simulink model "linearacc"  (R2020a)
settings: Solver=VariableStepAuto  StartTime=0.0  StopTime=10.0  RelTol=1e-3
undefined symbols (not defined in the file): Ax, Ay, Az, g, m
settings Model: Creator=Muni Kumar  LastModifiedBy=Muni Kumar

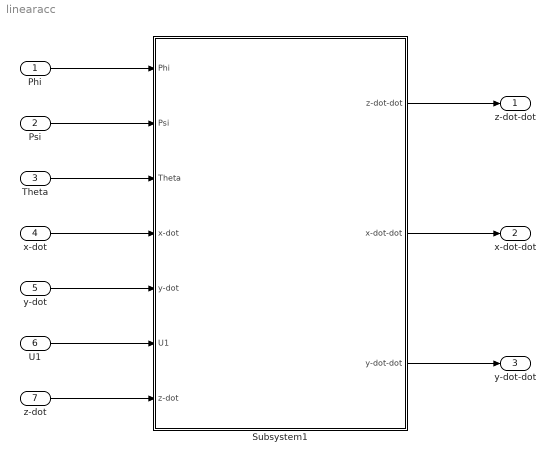
== system linearacc ==
  Phi : Inport
  Psi : Inport  Port=2
  Theta : Inport  Port=3
  x-dot : Inport  Port=4
  y-dot : Inport  Port=5
  U1 : Inport  Port=6
  z-dot : Inport  Port=7
  Subsystem1 : Subsystem
  z-dot-dot : Outport
  x-dot-dot : Outport  Port=2
  y-dot-dot : Outport  Port=3
  wires:
  Phi/1 -> Subsystem1/1(Phi)
  Psi/1 -> Subsystem1/2(Psi)
  Theta/1 -> Subsystem1/3(Theta)
  x-dot/1 -> Subsystem1/4(x-dot)
  U1/1 -> Subsystem1/6(U1)
  z-dot/1 -> Subsystem1/7(z-dot)
  Subsystem1/1(z-dot-dot) -> z-dot-dot/1
  Subsystem1/2(x-dot-dot) -> x-dot-dot/1
  Subsystem1/3(y-dot-dot) -> y-dot-dot/1
  y-dot/1 -> Subsystem1/5(y-dot)

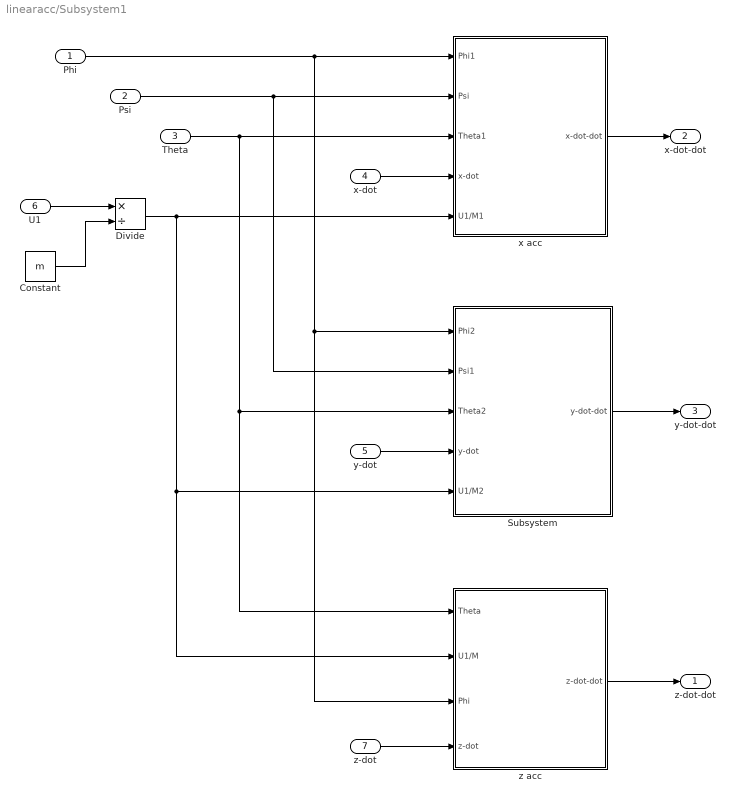
== system linearacc/Subsystem1 ==
  Phi : Inport
  Psi : Inport  Port=2
  Theta : Inport  Port=3
  x-dot : Inport  Port=4
  y-dot : Inport  Port=5
  U1 : Inport  Port=6
  z-dot : Inport  Port=7
  Constant : Constant  Value=m
  Divide : Product  Inputs=*/
  Subsystem : Subsystem
  x acc : Subsystem
  z acc : Subsystem
  z-dot-dot : Outport
  x-dot-dot : Outport  Port=2
  y-dot-dot : Outport  Port=3
  wires:
  Theta/1 -> x acc/3(Theta1), Subsystem/3(Theta2), z acc/1(Theta)
  Phi/1 -> Subsystem/1(Phi2), z acc/3(Phi), x acc/1(Phi1)
  Divide/1 -> Subsystem/5(U1/M2), z acc/2(U1/M), x acc/5(U1/M1)
  y-dot/1 -> Subsystem/4(y-dot)
  Constant/1 -> Divide/2
  Psi/1 -> Subsystem/2(Psi1), x acc/2(Psi)
  z-dot/1 -> z acc/4(z-dot)
  U1/1 -> Divide/1
  x-dot/1 -> x acc/4(x-dot)
  x acc/1(x-dot-dot) -> x-dot-dot/1
  z acc/1(z-dot-dot) -> z-dot-dot/1
  Subsystem/1(y-dot-dot) -> y-dot-dot/1

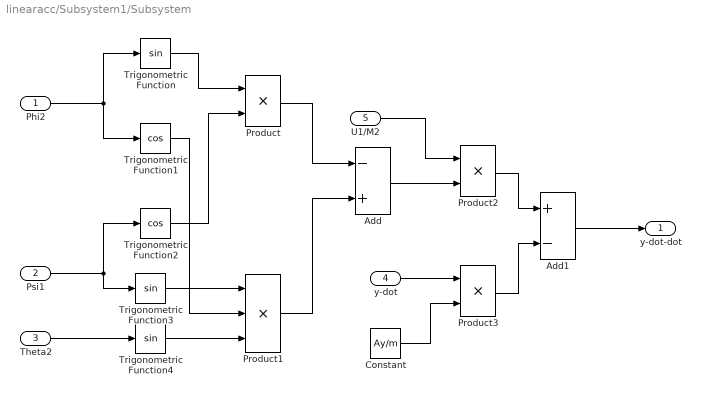
== system linearacc/Subsystem1/Subsystem ==
  Phi2 : Inport
  Psi1 : Inport  Port=2
  Theta2 : Inport  Port=3
  y-dot : Inport  Port=4
  U1/M2 : Inport  Port=5
  Add : Sum  Inputs=-+
  Add1 : Sum  Inputs=+-
  Constant : Constant  Value=Ay/m
  Product : Product
  Product1 : Product  Inputs=3
  Product2 : Product
  Product3 : Product
  Trigonometric Function : Trigonometry
  Trigonometric Function1 : Trigonometry  Operator=cos
  Trigonometric Function2 : Trigonometry  Operator=cos
  Trigonometric Function3 : Trigonometry
  Trigonometric Function4 : Trigonometry
  y-dot-dot : Outport
  wires:
  Phi2/1 -> Trigonometric Function1/1, Trigonometric Function/1
  Theta2/1 -> Trigonometric Function4/1
  Trigonometric Function1/1 -> Product1/2
  Add1/1 -> y-dot-dot/1
  Psi1/1 -> Trigonometric Function3/1, Trigonometric Function2/1
  Trigonometric Function4/1 -> Product1/3
  y-dot/1 -> Product3/1
  Product2/1 -> Add1/1
  U1/M2/1 -> Product2/1
  Product1/1 -> Add/2
  Add/1 -> Product2/2
  Constant/1 -> Product3/2
  Product/1 -> Add/1
  Trigonometric Function3/1 -> Product1/1
  Product3/1 -> Add1/2
  Trigonometric Function/1 -> Product/1
  Trigonometric Function2/1 -> Product/2

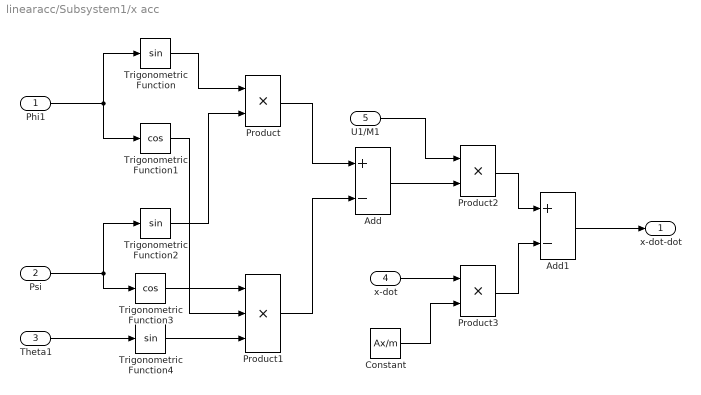
== system linearacc/Subsystem1/x acc ==
  Phi1 : Inport
  Psi : Inport  Port=2
  Theta1 : Inport  Port=3
  x-dot : Inport  Port=4
  U1/M1 : Inport  Port=5
  Add : Sum  Inputs=+-
  Add1 : Sum  Inputs=+-
  Constant : Constant  Value=Ax/m
  Product : Product
  Product1 : Product  Inputs=3
  Product2 : Product
  Product3 : Product
  Trigonometric Function : Trigonometry
  Trigonometric Function1 : Trigonometry  Operator=cos
  Trigonometric Function2 : Trigonometry
  Trigonometric Function3 : Trigonometry  Operator=cos
  Trigonometric Function4 : Trigonometry
  x-dot-dot : Outport
  wires:
  Phi1/1 -> Trigonometric Function1/1, Trigonometric Function/1
  x-dot/1 -> Product3/1
  Product3/1 -> Add1/2
  U1/M1/1 -> Product2/1
  Psi/1 -> Trigonometric Function3/1, Trigonometric Function2/1
  Trigonometric Function3/1 -> Product1/1
  Theta1/1 -> Trigonometric Function4/1
  Add/1 -> Product2/2
  Trigonometric Function1/1 -> Product1/2
  Trigonometric Function2/1 -> Product/2
  Product1/1 -> Add/2
  Product2/1 -> Add1/1
  Trigonometric Function/1 -> Product/1
  Trigonometric Function4/1 -> Product1/3
  Product/1 -> Add/1
  Constant/1 -> Product3/2
  Add1/1 -> x-dot-dot/1

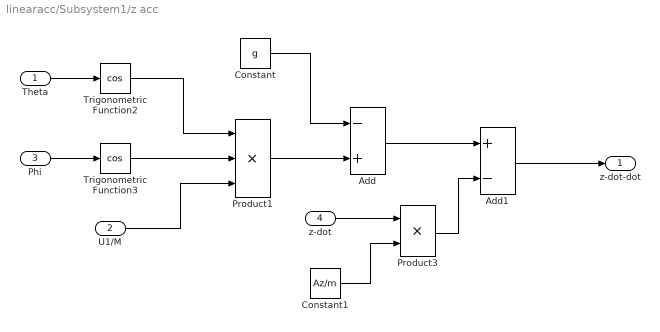
== system linearacc/Subsystem1/z acc ==
  Theta : Inport
  U1/M : Inport  Port=2
  Phi : Inport  Port=3
  z-dot : Inport  Port=4
  Add : Sum  Inputs=-+
  Add1 : Sum  Inputs=+-
  Constant : Constant  Value=g
  Constant1 : Constant  Value=Az/m
  Product1 : Product  Inputs=3
  Product3 : Product
  Trigonometric Function2 : Trigonometry  Operator=cos
  Trigonometric Function3 : Trigonometry  Operator=cos
  z-dot-dot : Outport
  wires:
  Phi/1 -> Trigonometric Function3/1
  Product3/1 -> Add1/2
  U1/M/1 -> Product1/3
  Theta/1 -> Trigonometric Function2/1
  Add/1 -> Add1/1
  Product1/1 -> Add/2
  Add1/1 -> z-dot-dot/1
  Constant1/1 -> Product3/2
  z-dot/1 -> Product3/1
  Trigonometric Function3/1 -> Product1/2
  Constant/1 -> Add/1
  Trigonometric Function2/1 -> Product1/1
